simulink model "msample_time_precision"  (Simulink 6.3)
settings: Solver=ode4  StartTime=0.0  StopTime=10.0  FixedStep=1/300  RelTol=1e-3
settings Model: Creator=wsyed  LastModifiedBy=awarlock  ExtModeAutoUpdateStatusClock=off  StrictBusMsg=ErrorLevel1
settings MATStruct: SampleTime=0.00167  Offset=0  Priority=[20.0]
settings OptimizationCC: InlineInvariantSignals=on

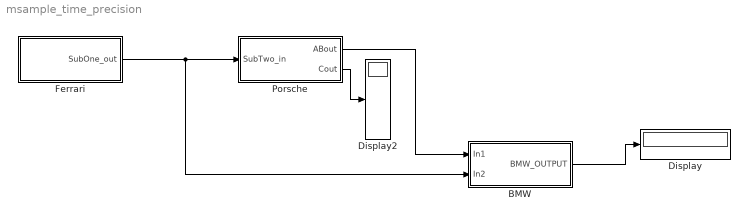
== system msample_time_precision ==
  BMW : Subsystem  TreatAsAtomicUnit=on
  Display : Display
  Display2 : Display
  Ferrari : Subsystem  TreatAsAtomicUnit=on
  Porsche : Subsystem  TreatAsAtomicUnit=on
  wires:
  Ferrari/1(SubOne_out) -> Porsche/1(SubTwo_in), BMW/2(In2)
  Porsche/1(ABout) -> BMW/1(In1)
  BMW/1(BMW_OUTPUT) -> Display/1
  Porsche/2(Cout) -> Display2/1

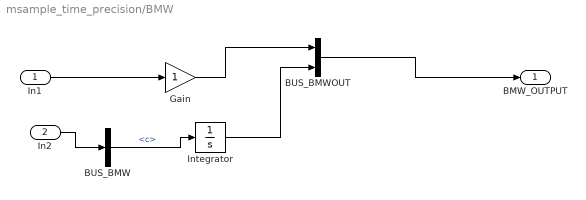
== system msample_time_precision/BMW ==
  In1 : Inport  Port=1  LatchInput=off
  In2 : Inport  Port=2  LatchInput=off
  BUS_BMW : BusSelector  OutputSignals=c
  BUS_BMWOUT : BusCreator  Inputs=2
  Gain : Gain
  Integrator : Integrator
  BMW_OUTPUT : Outport
  wires:
  In1/1 -> Gain/1
  In2/1 -> BUS_BMW/1
  BUS_BMW/1 -> Integrator/1  "<c>"
  Gain/1 -> BUS_BMWOUT/1
  Integrator/1 -> BUS_BMWOUT/2
  BUS_BMWOUT/1 -> BMW_OUTPUT/1

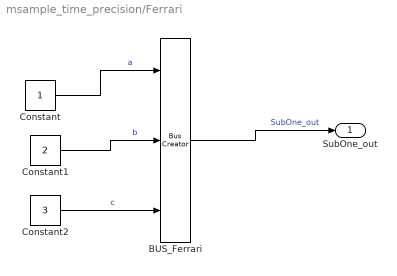
== system msample_time_precision/Ferrari ==
  BUS_Ferrari : BusCreator  Inputs=3
  Constant : Constant
  Constant1 : Constant  Value=2
  Constant2 : Constant  Value=3
  SubOne_out : Outport
  wires:
  Constant/1 -> BUS_Ferrari/1  "a"
  Constant1/1 -> BUS_Ferrari/2  "b"
  Constant2/1 -> BUS_Ferrari/3  "c"
  BUS_Ferrari/1 -> SubOne_out/1  "SubOne_out"

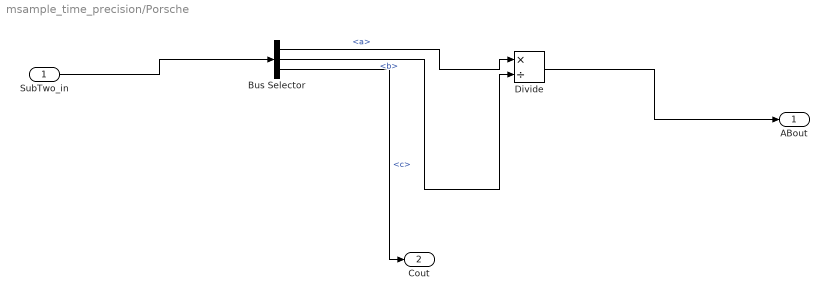
== system msample_time_precision/Porsche ==
  SubTwo_in : Inport  Port=1  LatchInput=off
  Bus Selector : BusSelector  OutputSignals=a,b,c
  Divide : Product  Inputs=*/  OutScaling=2^-10
  ABout : Outport
  Cout : Outport  Port=2
  wires:
  SubTwo_in/1 -> Bus Selector/1
  Bus Selector/1 -> Divide/1  "<a>"
  Bus Selector/2 -> Divide/2  "<b>"
  Divide/1 -> ABout/1
  Bus Selector/3 -> Cout/1  "<c>"
